simulink model "Primerpunto"  (R2015b)
settings: Solver=VariableStepAuto  StartTime=0.0  StopTime=1  RelTol=1e-3
libraries: commutil2 x4, commsrccod2 x2, dspquant2 x2, dspsrcs4 x1, dspvision x1
settings Model: Creator=pc  LastModifiedBy=pc

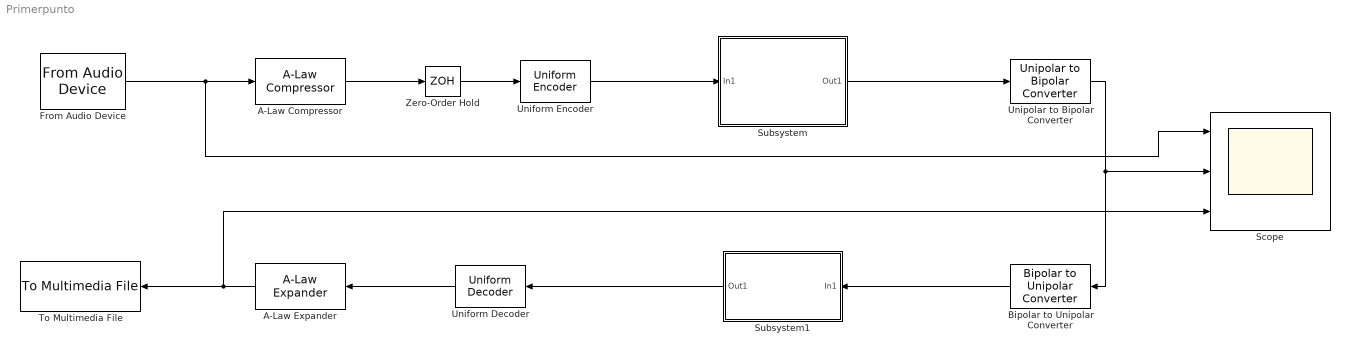
== system Primerpunto ==
  A-Law Compressor : commsrccod2/A-Law Compressor  A=87.6  V=20
  A-Law Expander : commsrccod2/A-Law Expander  A=87.6  V=20
  Bipolar to Unipolar Converter : commutil2/Bipolar to Unipolar Converter  M=8  polarity=Positive  dataType=int8
  From Audio Device : dspsrcs4/From Audio Device  deviceName=Default  numChannels=1  sampleRate=44100  deviceDatatype=Determine from output data type  autoBufferSize=on  bufferSize=4096  queueDuration=0.1  frameSize=1  outputDatatype=double  defaultInputChannelMapping=on  inputChannelMapping=1:2  outputNumOverrunSamples=off  OutputFrames=off
  Scope : Scope  NumInputPorts=3
  Subsystem : Subsystem
  Subsystem1 : Subsystem
  To Multimedia File : dspvision/To Multimedia File  outputFilename=output.wav  streamSelection=Audio only  videoCompressor=None (uncompressed)  audioCompressor=None (uncompressed)  imagePorts=Separate color signals  fileType=WAV  audioDatatype=16-bit integer  fourcc=RGB  videoQuality=75  mj2000CompFactor=10
  Uniform Decoder : dspquant2/Uniform Decoder  peak=20  bits=8  overflowMode=Saturate  otype=Double
  Uniform Encoder : dspquant2/Uniform Encoder  peak=20  bits=8  otype=Unsigned integer
  Unipolar to Bipolar Converter : commutil2/Unipolar to Bipolar Converter  M=8  polarity=Positive  dataType=Inherit via internal rule
  Zero-Order Hold : ZeroOrderHold  SampleTime=1/(8*4000)
  wires:
  Zero-Order Hold/1 -> Uniform Encoder/1
  Unipolar to Bipolar Converter/1 -> Scope/2, Bipolar to Unipolar Converter/1
  A-Law Expander/1 -> Scope/3, To Multimedia File/1
  From Audio Device/1 -> Scope/1, A-Law Compressor/1
  A-Law Compressor/1 -> Zero-Order Hold/1
  Uniform Decoder/1 -> A-Law Expander/1
  Uniform Encoder/1 -> Subsystem/1(In1)
  Subsystem/1(Out1) -> Unipolar to Bipolar Converter/1
  Bipolar to Unipolar Converter/1 -> Subsystem1/1(In1)
  Subsystem1/1(Out1) -> Uniform Decoder/1

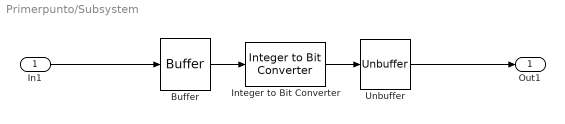
== system Primerpunto/Subsystem ==
  In1 : Inport
  Buffer : Buffer  N=1  TreatMby1Signals=One channel  OutputFrames=off
  Integer to Bit Converter : commutil2/Integer to Bit Converter  nbits=8  signedInputValues=Signed  bitOrder=MSB first  outDtype=Inherit via internal rule
  Unbuffer : Unbuffer  ic=3  SampleBasedProcessing=Same as frame based
  Out1 : Outport
  wires:
  Integer to Bit Converter/1 -> Unbuffer/1
  Unbuffer/1 -> Out1/1
  Buffer/1 -> Integer to Bit Converter/1
  In1/1 -> Buffer/1

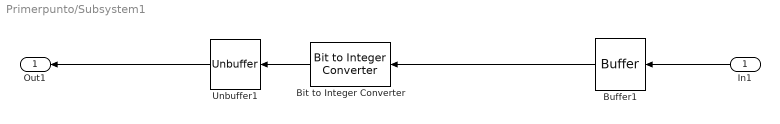
== system Primerpunto/Subsystem1 ==
  In1 : Inport
  Bit to Integer Converter : commutil2/Bit to Integer Converter  nbits=3  bitOrder=MSB first  signedOutputValues=Unsigned  outDtype=Inherit via internal rule  outDtypeSigned=Inherit via internal rule
  Buffer1 : Buffer  N=3  TreatMby1Signals=One channel  OutputFrames=off
  Unbuffer1 : Unbuffer  SampleBasedProcessing=Same as frame based
  Out1 : Outport
  wires:
  Buffer1/1 -> Bit to Integer Converter/1
  In1/1 -> Buffer1/1
  Bit to Integer Converter/1 -> Unbuffer1/1
  Unbuffer1/1 -> Out1/1
